simulink model "Eve_v2_Simulator_inout_linss"  (R2017b)
settings: Solver=VariableStepAuto  StartTime=0.0  StopTime=sTime  FixedStep=delta_t  RelTol=1e-12
values from neighbouring files (symbols this model uses):
  delta_t = ssmodelo.Ts    [todorov_getgains_p.m]
undefined symbols (not defined in the file or in its folder): alpha1, alpha2, DiscIntNeverNeededParam, qy, y_0
libraries: aerolibutil x4, sharedutil x3, dspmathops x2, discretizing x1, simulink x1
settings Model: Creator=carlos  LastModifiedBy=ruiem
settings ModelReferenceCC: ModelReferenceNumInstancesAllowed=Single
settings CodeAppCC: StateflowObjectComments=on

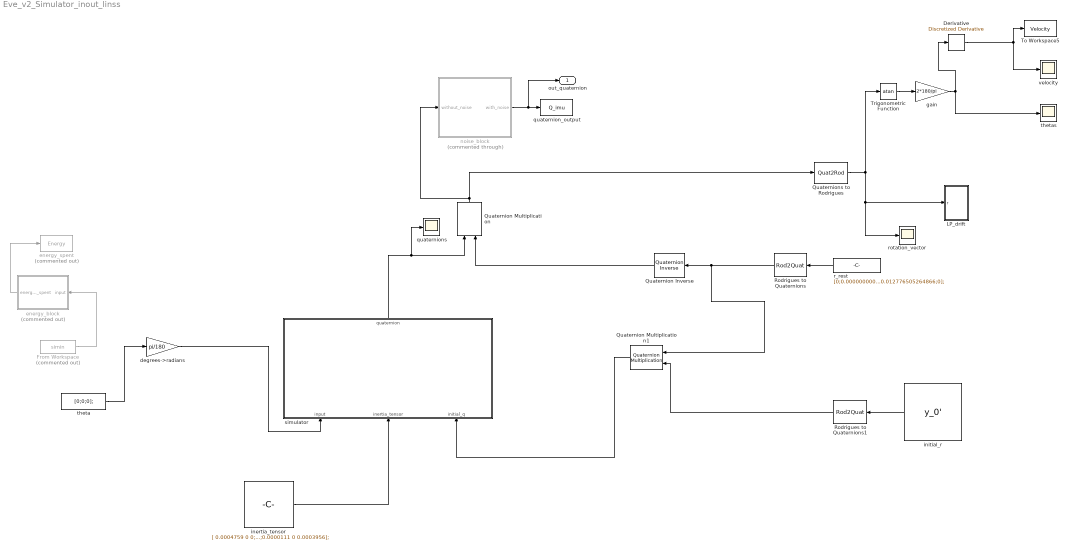
== system Eve_v2_Simulator_inout_linss ==
  Derivative : discretizing/Discretized Derivative  method=tustin  SampleTime=0.001  Wc=1
  From Workspace : FromWorkspace  Commented=on  VariableName=simin  SampleTime=0.01
  LP_drift : Subsystem
  Quaternion Inverse : aerolibutil/Quaternion Inverse
      settings: SourceProductName=Aerospace Blockset
  Quaternion Multiplication : aerolibutil/Quaternion Multiplication
  Quaternion Multiplication1 : aerolibutil/Quaternion Multiplication
  Quaternions to Rodrigues : Quat2Rod
  Rodrigues to Quaternions : Rod2Quat
  Rodrigues to Quaternions1 : Rod2Quat
  To Workspace5 : ToWorkspace  VariableName=Velocity  SaveFormat=Timeseries  SampleTime=0.01
  Trigonometric Function : Trigonometry  Operator=atan
  degrees->radians : Gain  Gain=pi/180
  energy_block : Subsystem  Commented=on
  energy_spent : ToWorkspace  Commented=on  VariableName=Energy  SaveFormat=Timeseries  SampleTime=0.01
  gain : Gain  Gain=2*180/pi
  inertia_tensor : Constant  Value=[ 0.0004759 0 0;0 0.0004759 0;0 0 0.0004759]; %[ 0.0004759 -0.0000001 0.0000111;-0.0000001 0.0004316 0;0.0000111 0 0.0003956];
  initial_r : Constant  Value=y_0'
  noise_block : Subsystem  Commented=through
  quaternion_output : ToWorkspace  VariableName=Q_imu  SaveFormat=Timeseries  SampleTime=delta_t
  quaternions : Scope
  r_rest : Constant  Value=[0;0.0000000000000001;0] %[0;-0.012776505264866;0];
  rotation_vector : Scope
  simulator : Subsystem
  theta : Constant  Value=[0;0;0];
  thetas : Scope
  velocity : Scope
  out_quaternion : Outport
  wires:
  Quaternions to Rodrigues/1 -> rotation_vector/1, LP_drift/1(r), Trigonometric Function/1
  Trigonometric Function/1 -> gain/1
  gain/1 -> Derivative/1, thetas/1
  From Workspace/1 -> energy_block/1(input)
  Rodrigues to Quaternions/1 -> Quaternion Inverse/1, Quaternion Multiplication1/1
  Quaternion Multiplication/1 -> Quaternions to Rodrigues/1, noise_block/1(without_noise)
  initial_r/1 -> Rodrigues to Quaternions1/1
  Quaternion Inverse/1 -> Quaternion Multiplication/2
  Derivative/1 -> To Workspace5/1, velocity/1
  Rodrigues to Quaternions1/1 -> Quaternion Multiplication1/2
  r_rest/1 -> Rodrigues to Quaternions/1
  noise_block/1(with_noise) -> out_quaternion/1, quaternion_output/1
  energy_block/1(energy_spent) -> energy_spent/1
  simulator/1(quaternion) -> Quaternion Multiplication/1, quaternions/1
  degrees->radians/1 -> simulator/1(input)
  Quaternion Multiplication1/1 -> simulator/3(initial_q)
  inertia_tensor/1 -> simulator/2(inertia_tensor)
  theta/1 -> degrees->radians/1

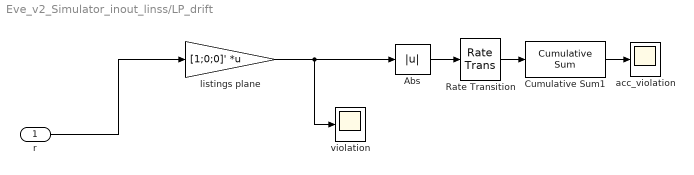
== system Eve_v2_Simulator_inout_linss/LP_drift ==
  r : Inport
  Abs : Abs
  Cumulative Sum1 : dspmathops/Cumulative Sum  dim=Channels (running sum)  InputProcessing=Columns as channels (frame based)  reset_popup=None  outputDataTypeStr=Inherit: Same as accumulator  outputLastDataTypeStr=Inherit: Same as accumulator  outputMin=[]  outputMax=[]  roundingMode=Floor  overflowMode=off
      settings: SourceProductName=DSP System Toolbox
  Rate Transition : RateTransition  OutPortSampleTime=0.01
  acc_violation : Scope
  listings plane : Gain  Gain=[1;0;0]'  Multiplication=Matrix(K*u)
  violation : Scope
  wires:
  Abs/1 -> Rate Transition/1
  Rate Transition/1 -> Cumulative Sum1/1
  Cumulative Sum1/1 -> acc_violation/1
  listings plane/1 -> violation/1, Abs/1
  r/1 -> listings plane/1

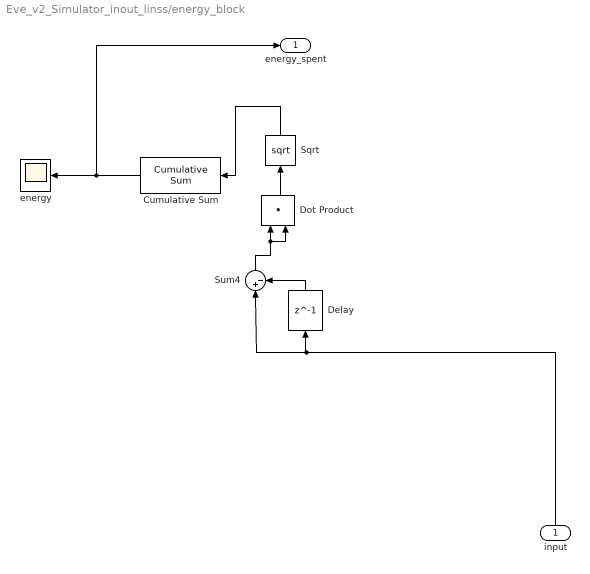
== system Eve_v2_Simulator_inout_linss/energy_block ==
  input : Inport
  Cumulative Sum : dspmathops/Cumulative Sum  dim=Channels (running sum)  InputProcessing=Columns as channels (frame based)  reset_popup=None  outputDataTypeStr=Inherit: Same as accumulator  outputLastDataTypeStr=Inherit: Same as accumulator  outputMin=[]  outputMax=[]  roundingMode=Floor  overflowMode=off
      settings: SourceProductName=DSP System Toolbox
  Delay : Delay  DelayLength=1  InitialCondition=0  SampleTime=0.01
  Dot Product : DotProduct  InputSameDT=on  OutDataTypeStr=Inherit: Inherit via internal rule
  Sqrt : Sqrt  SaturateOnIntegerOverflow=on
  Sum4 : Sum  Inputs=|+-
  energy : Scope
  energy_spent : Outport
  wires:
  Sqrt/1 -> Cumulative Sum/1
  input/1 -> Sum4/1, Delay/1
  Delay/1 -> Sum4/2
  Sum4/1 -> Dot Product/2, Dot Product/1
  Dot Product/1 -> Sqrt/1
  Cumulative Sum/1 -> energy_spent/1, energy/1

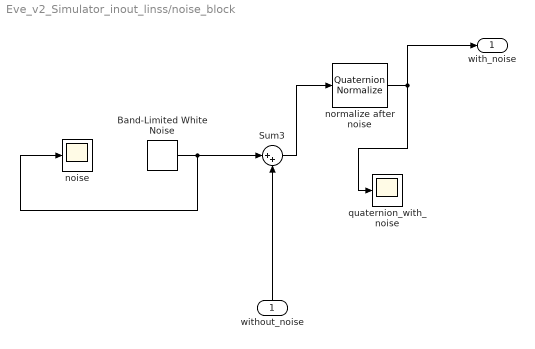
== system Eve_v2_Simulator_inout_linss/noise_block ==
  without_noise : Inport
  Band-Limited White Noise : simulink/Sources/Band-Limited White Noise  Cov=[0]  Ts=delta_t  seed=[23341]
  Sum3 : Sum  Inputs=|++
  noise : Scope
  normalize after noise : sharedutil/Quaternion Normalize
      settings: SourceProductName=Aerospace Blockset  SourceProductBaseCode=AE
  quaternion_with_noise : Scope
  with_noise : Outport
  wires:
  Band-Limited White Noise/1 -> noise/1, Sum3/1
  Sum3/1 -> normalize after noise/1
  normalize after noise/1 -> with_noise/1, quaternion_with_noise/1
  without_noise/1 -> Sum3/2

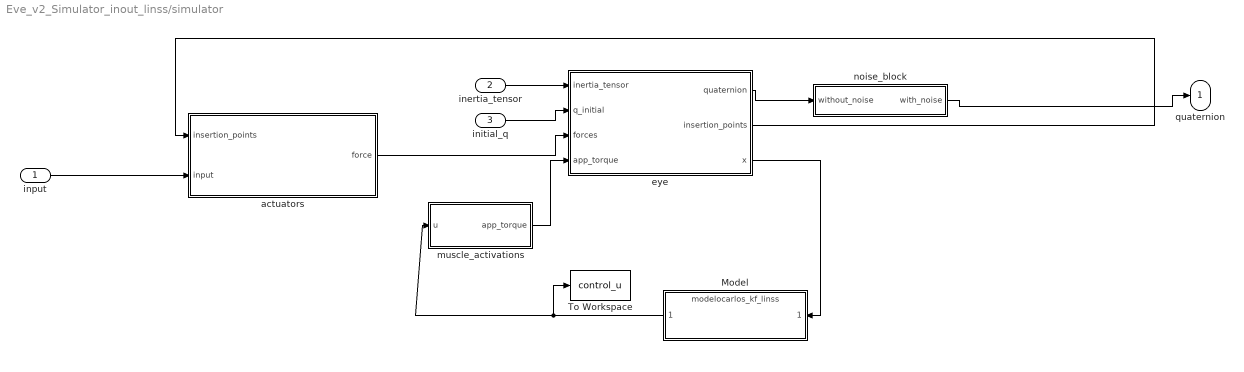
== system Eve_v2_Simulator_inout_linss/simulator ==
  input : Inport
  inertia_tensor : Inport  Port=2
  initial_q : Inport  Port=3
  Model : ModelReference  ModelNameDialog=modelocarlos_kf_linss.slx  SimulationMode=Normal  ModelReferenceVersion=1.230
  To Workspace : ToWorkspace  VariableName=control_u  SampleTime=-1
  actuators : Subsystem
  eye : Subsystem
  muscle_activations : Subsystem
  noise_block : Subsystem
  quaternion : Outport
  wires:
  input/1 -> actuators/2(input)
  inertia_tensor/1 -> eye/1(inertia_tensor)
  initial_q/1 -> eye/2(q_initial)
  actuators/1(force) -> eye/3(forces)
  eye/2(insertion_points) -> actuators/1(insertion_points)
  muscle_activations/1(app_torque) -> eye/4(app_torque)
  eye/1(quaternion) -> noise_block/1(without_noise)
  noise_block/1(with_noise) -> quaternion/1
  eye/3(x) -> Model/1
  Model/1 -> To Workspace/1, muscle_activations/1(u)

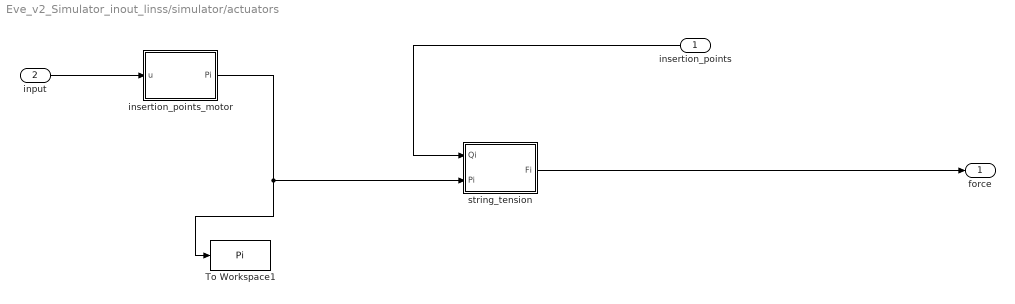
== system Eve_v2_Simulator_inout_linss/simulator/actuators ==
  insertion_points : Inport
  input : Inport  Port=2
  To Workspace1 : ToWorkspace  VariableName=Pi  SaveFormat=Timeseries  SampleTime=-1
  insertion_points_motor : MATLAB Function  TreatAsAtomicUnit=on
  string_tension : MATLAB Function  TreatAsAtomicUnit=on
  force : Outport
  wires:
  input/1 -> insertion_points_motor/1(u)
  insertion_points_motor/1(Pi) -> To Workspace1/1, string_tension/2(Pi)
  string_tension/1(Fi) -> force/1
  insertion_points/1 -> string_tension/1(Qi)

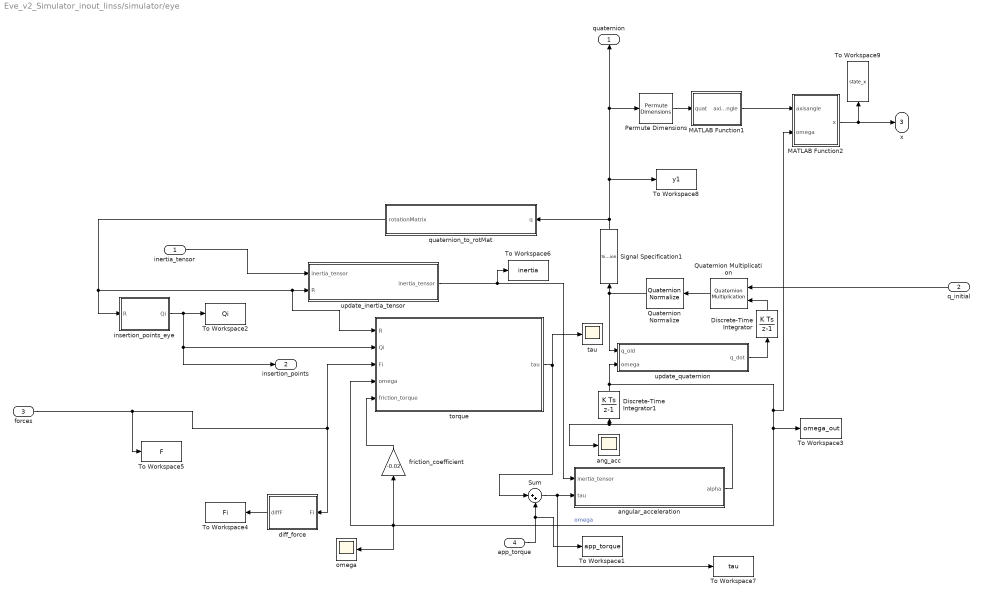
== system Eve_v2_Simulator_inout_linss/simulator/eye ==
  inertia_tensor : Inport
  q_initial : Inport  Port=2
  forces : Inport  Port=3
  app_torque : Inport  Port=4
  Discrete-Time Integrator : DiscreteIntegrator  InitialCondition=[1 0 0 0]  InitialConditionSetting=State (most efficient)  SampleTime=-1  ICPrevOutput=DiscIntNeverNeededParam  ICPrevScaledInput=DiscIntNeverNeededParam
  Discrete-Time Integrator1 : DiscreteIntegrator  InitialConditionSetting=State (most efficient)  SampleTime=-1  ICPrevOutput=DiscIntNeverNeededParam  ICPrevScaledInput=DiscIntNeverNeededParam
  MATLAB Function1 : MATLAB Function  TreatAsAtomicUnit=on
  MATLAB Function2 : MATLAB Function  TreatAsAtomicUnit=on
  Permute Dimensions : PermuteDimensions
  Quaternion Multiplication : aerolibutil/Quaternion Multiplication
  Quaternion Normalize : sharedutil/Quaternion Normalize
      settings: SourceProductName=Aerospace Blockset  SourceProductBaseCode=AE
  Signal Specification1 : SignalSpecification  Dimensions=[1 4]
  Sum : Sum  Inputs=|++
  To Workspace1 : ToWorkspace  VariableName=app_torque  SampleTime=delta_t
  To Workspace2 : ToWorkspace  VariableName=Qi  SaveFormat=Timeseries  SampleTime=-1
  To Workspace3 : ToWorkspace  VariableName=omega_out  SampleTime=-1
  To Workspace4 : ToWorkspace  VariableName=Fi  SaveFormat=Timeseries  SampleTime=0.1
  To Workspace5 : ToWorkspace  VariableName=F  SampleTime=delta_t
  To Workspace6 : ToWorkspace  VariableName=inertia  SampleTime=delta_t
  To Workspace7 : ToWorkspace  VariableName=tau  SampleTime=delta_t
  To Workspace8 : ToWorkspace  VariableName=y1  SampleTime=delta_t
  To Workspace9 : ToWorkspace  VariableName=state_x  SampleTime=delta_t
  ang_acc : Scope
  angular_acceleration : MATLAB Function  TreatAsAtomicUnit=on
  diff_force : MATLAB Function  TreatAsAtomicUnit=on
  friction_coefficient : Gain  Gain=-0.02
  insertion_points_eye : MATLAB Function  TreatAsAtomicUnit=on
  omega : Scope
  quaternion_to_rotMat : MATLAB Function  TreatAsAtomicUnit=on
  tau : Scope
  torque : MATLAB Function  TreatAsAtomicUnit=on
  update_inertia_tensor : MATLAB Function  TreatAsAtomicUnit=on
  update_quaternion : MATLAB Function  TreatAsAtomicUnit=on
  quaternion : Outport  PortDimensions=[1 4]
  insertion_points : Outport  Port=2
  x : Outport  Port=3
  wires:
  q_initial/1 -> Quaternion Multiplication/1
  Quaternion Normalize/1 -> Signal Specification1/1, update_quaternion/1(q_old)
  diff_force/1(diffF) -> To Workspace4/1
  angular_acceleration/1(alpha) -> Discrete-Time Integrator1/1, ang_acc/1
  quaternion_to_rotMat/1(rotationMatrix) -> torque/1(R), update_inertia_tensor/2(R), insertion_points_eye/1(R)
  inertia_tensor/1 -> update_inertia_tensor/1("inertia_tensor ")
  insertion_points_eye/1(Qi) -> insertion_points/1, torque/2(Qi), To Workspace2/1
  update_inertia_tensor/1(inertia_tensor) -> To Workspace6/1, angular_acceleration/1(inertia_tensor)
  friction_coefficient/1 -> torque/5(friction_torque)
  Discrete-Time Integrator1/1 -> update_quaternion/2(omega), MATLAB Function2/2(omega), To Workspace3/1, omega/1, torque/4(omega), friction_coefficient/1  "omega"
  forces/1 -> To Workspace5/1, torque/3(Fi), diff_force/1(Fi)
  Quaternion Multiplication/1 -> Quaternion Normalize/1
  torque/1(tau) -> tau/1, Sum/1
  app_torque/1 -> Sum/2, To Workspace1/1
  Sum/1 -> To Workspace7/1, angular_acceleration/2(tau)
  update_quaternion/1(q_dot) -> Discrete-Time Integrator/1
  Discrete-Time Integrator/1 -> Quaternion Multiplication/2
  MATLAB Function1/1(axisangle) -> MATLAB Function2/1(axisangle)
  MATLAB Function2/1(x) -> x/1, To Workspace9/1
  Permute Dimensions/1 -> MATLAB Function1/1(quat)
  Signal Specification1/1 -> To Workspace8/1, Permute Dimensions/1, quaternion/1, quaternion_to_rotMat/1(q)

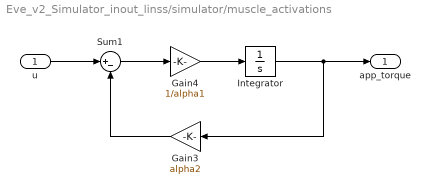
== system Eve_v2_Simulator_inout_linss/simulator/muscle_activations ==
  u : Inport
  Gain3 : Gain  Gain=alpha2
  Gain4 : Gain  Gain=1/alpha1
  Integrator : Integrator
  Sum1 : Sum  Inputs=|+-
  app_torque : Outport
  wires:
  Integrator/1 -> app_torque/1, Gain3/1
  Gain3/1 -> Sum1/2
  Sum1/1 -> Gain4/1
  Gain4/1 -> Integrator/1
  u/1 -> Sum1/1

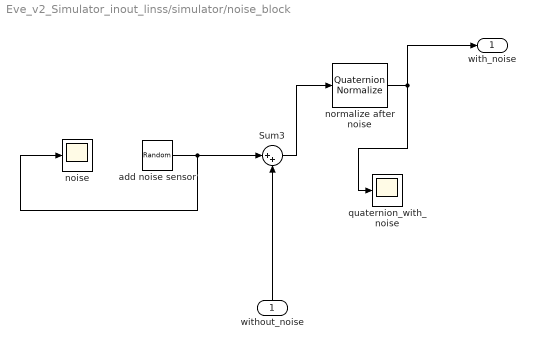
== system Eve_v2_Simulator_inout_linss/simulator/noise_block ==
  without_noise : Inport  PortDimensions=4
  Sum3 : Sum  Inputs=|++
  add noise sensor : RandomNumber  Variance=qy^2  SampleTime=delta_t
  noise : Scope
  normalize after noise : sharedutil/Quaternion Normalize
      settings: SourceProductName=Aerospace Blockset  SourceProductBaseCode=AE
  quaternion_with_noise : Scope
  with_noise : Outport  PortDimensions=4
  wires:
  add noise sensor/1 -> noise/1, Sum3/1
  Sum3/1 -> normalize after noise/1
  normalize after noise/1 -> with_noise/1, quaternion_with_noise/1
  without_noise/1 -> Sum3/2

== matlab function Eve_v2_Simulator_inout_linss/simulator/eye/update_quaternion ==
  data: q_old input; q_dot output; omega input
function q_dot = update_quaternion(q_old, omega)

%q_dot = zeros(1,4);
q_dot = 1/2*quatmultiply([0 omega(1) omega(2) omega(3)], q_old);

== matlab function Eve_v2_Simulator_inout_linss/simulator/eye/quaternion_to_rotMat ==
  data: q input; rotationMatrix output
function rotationMatrix = rotMat(q)

rotationMatrix = zeros(3,3);

s = norm(q)^-2;

rotationMatrix(1,1) = 1-2*s*(q(3)*q(3)+q(4)*q(4));
rotationMatrix(1,2) = 2*s*(q(3)*q(2)-q(4)*q(1));
rotationMatrix(1,3) = 2*s*(q(2)*q(4)+q(1)*q(3));
rotationMatrix(2,1) = 2*s*(q(3)*q(2)+q(4)*q(1));
rotationMatrix(2,2) = 1-2*s*(q(2)*q(2)+q(4)*q(4));
rotationMatrix(2,3) = 2*s*(q(3)*q(4)-q(1)*q(2));
rotationMatrix(3,1) = 2*s*(q(2)*q(4)-q(3)*q(1));
rotationMatrix(3,2) = 2*s*(q(3)*q(4)+q(2)*q(1));
rotationMatrix(3,3) = 1-2*(q(2)*q(2)+q(3)*q(3));

== matlab function Eve_v2_Simulator_inout_linss/simulator/actuators/insertion_points_motor ==
  data: u input; Pi output
    function Pi = get_Pi(u)

% get new P
P1 = [-0.436 - 0.1*sin(u(1)); -0.0835; 0.021 + 0.1*cos(u(1))];
P2 = [-0.436 + 0.1*sin(u(1)); -0.0835; 0.021 - 0.1*cos(u(1))];

P3 = [-0.323 - 0.140*sin(u(2)); -0.140*cos(u(2)); 0.0475];%-0.323
P4 = [-0.323 + 0.140*sin(u(2)); 0.140*cos(u(2)); 0.0475];%-0.323

P5 = [-0.436 + 0.1*sin(u(3)); 0.0835; 0.021 + 0.1*cos(u(3))];
P6 = [-0.436 - 0.1*sin(u(3)); 0.0835; 0.021 - 0.1*cos(u(3))];

% concatenate
Pi = [P1 P2 P3 P4 P5 P6];

== matlab function Eve_v2_Simulator_inout_linss/simulator/eye/insertion_points_eye ==
  data: R input; Qi output
function Qi = get_Qi(R)

% get new Q
Q1_0 = [-0.007; 0.05302; 0.05302];
Q2_0 = [-0.007; 0.05302; -0.05302];

Q3_0 = [-0.007; -0.07498; 0];
Q4_0 = [-0.007; 0.07498; 0];

Q5_0 = [-0.007; -0.05302; 0.05302];
Q6_0 = [-0.007; -0.05302; -0.05302];

Q1 = R*Q1_0;
Q2 = R*Q2_0;
Q3 = R*Q3_0;
Q4 = R*Q4_0;
Q5 = R*Q5_0;
Q6 = R*Q6_0;

% concatenate
Qi = [Q1 Q2 Q3 Q4 Q5 Q6];

== matlab function Eve_v2_Simulator_inout_linss/simulator/actuators/string_tension ==
  data: Qi input; Pi input; Fi output
function Fi = get_Fi(Qi, Pi)

% constants
k = 6;

l1_0 = 34 * 10^-2;
l2_0 = 36 * 10^-2;
l3_0 = 24 * 10^-2;
l4_0 = 24 * 10^-2;
l5_0 = 34 * 10^-2;
l6_0 = 36 * 10^-2;

li_0 = [l1_0 l2_0 l3_0 l4_0 l5_0 l6_0];

% connection points
X1 = [-0.2055; 0; 0.0525];
X2 = [-0.2055; 0; -0.0525];

X5 = X1;
X6 = X2;
%X5 = [-0.2055; 0; 0.0625];
%X6 = [-0.2055; 0; -0.0625];

% intermediate insertion points
Xi = [X1 X2 Qi(:,3) Qi(:,4) X5 X6];

% intermediate string direction points
Yi = [X1 X2 Pi(:,3) Pi(:,4) X5 X6];

% get string length
% l1 = norm(Pi(:,1) - X1) + norm(X1 - Qi(:,1));
% l2 = norm(Pi(:,2) - X2) + norm(X2 - Qi(:,2));
% l3 = norm(Pi(:,3) - Qi(:,3));
% l4 = norm(Pi(:,4) - Qi(:,4));
% l5 = norm(Pi(:,5) - X5) + norm(X5 - Qi(:,5));
% l6 = norm(Pi(:,6) - X6) + norm(X6 - Qi(:,6));

li = zeros(1,6);

for i=1:6
    li(i) = norm(Pi(:,i) - Xi(:,i)) + norm(Xi(:,i) - Qi(:,i));
end


% string directions
% d1 = (X1 - Q1)/norm(X1 - Q1);
% d2 = (X2 - Q2)/norm(X2 - Q2);
% d3 = (P3 - Q3)/norm(P3 - Q3);
% d4 = (P4 - Q4)/norm(P4 - Q4);
% d5 = (X5 - Q5)/norm(X5 - Q5);
% d6 = (X6 - Q6)/norm(X6 - Q6);

di = zeros(3,6);

for i=1:6
    di(:,i) = (Yi(:,i) - Qi(:,i))/norm(Yi(:,i) - Qi(:,i));
end


Fi = zeros(3,6);

for i=1:6
    Fi(:,i) = k/li_0(i)*max((li(i)-li_0(i)),0) * di(:,i);
end

% F1 = k/l1_0*max((l1-l1_0),0) * d1;
% F2 = k/l2_0*max((l2-l2_0),0) * d2;
% F3 = k/l3_0*max((l3-l3_0),0) * d3;
% F4 = k/l4_0*max((l4-l4_0),0) * d4;
% F5 = k/l5_0*max((l5-l5_0),0) * d5;
% F6 = k/l6_0*max((l6-l6_0),0) * d6;

% concatenate
% Fi = [F1 F2 F3 F4 F5 F6];

== matlab function Eve_v2_Simulator_inout_linss/simulator/eye/diff_force ==
  data: Fi input; diffF output
function diffF = get_diffF(Fi)

diffF = 0;

for i=2:2:size(Fi,2)
    diffF = diffF + abs(norm(Fi(:,i-1))-norm(Fi(:,i)));
end

== matlab function Eve_v2_Simulator_inout_linss/simulator/eye/torque ==
  data: R input; Qi input; Fi input; tau output; omega input; friction_torque input
function tau = get_torque(R, Qi, Fi, omega, friction_torque)

tau = zeros(3,1);

for i=1:6
    tau = tau + cross(Qi(:,i), Fi(:,i));
end

center_mass = R*[0.02; 0; 0]; % center of mass
mass = 0.248; % mass in kg
Fg = mass*[0; 0; -9.8];
taug = cross(center_mass, Fg);

tau = tau + taug;

tau = tau + friction_torque;
%tau=zeros(3,1); 
% ntau = norm(tau);
static_friction_torque = 0*0.006;
if norm(omega) < 0.00001
    if norm(tau) < static_friction_torque
        tau = zeros(3,1);
    end
end

== matlab function Eve_v2_Simulator_inout_linss/simulator/eye/angular_acceleration ==
  data: inertia_tensor input; tau input; alpha output
function alpha = get_ang_acc(inertia_tensor, tau)

alpha = zeros(3,1);
alpha = inertia_tensor\tau;

== matlab function Eve_v2_Simulator_inout_linss/simulator/eye/update_inertia_tensor ==
  data: inertia_tensor input; inertia_tensor output; R input
function inertia_tensor = update_inertia_tensor(inertia_tensor, R)

% transform inertia tensor to world reference frame
inertia_tensor = R'*inertia_tensor*R;

== matlab function Eve_v2_Simulator_inout_linss/simulator/eye/MATLAB Function2 ==
  data: axisangle input; x output; omega input
function x = concat_state(axisangle, omega)

x=[axisangle; omega];

== matlab function Eve_v2_Simulator_inout_linss/simulator/eye/MATLAB Function1 ==
  data: quat input; axisangle output
function axisangle = fcn(quat)

axang=quat2axang(quat');
axisangle=axang(1:3)'*axang(4);
%eul=rotvec(quat);
% aux=(quat./quat(1))';
% eul=aux(1,2:4)';
